simulink library "F_Line_block"  (R2018a)
settings: Solver=VariableStepAuto  StartTime=0.0  StopTime=10.0  RelTol=1e-3  EnableMultiTasking=on
settings Model: Creator=altari  LastModifiedBy=DW
settings DataIOCC: LimitDataPoints=on
settings OptimizationCC: LifeSpan=inf
settings DebuggingCC: AllowSymbolicDim=off  SFUnexpectedBacktrackingDiag=warning  SFNoUnconditionalDefaultTransitionDiag=warning  SFExecutionAtInitializationDiag=none
settings ModelReferenceCC: PropagateSignalLabelsOutOfModel=off
settings CodeAppCC: StateflowObjectComments=on
settings GRTTargetCC: TargetLangStandard=C89/C90 (ANSI)
settings ConfigComp: CovMetricSettings=dw  CovHtmlReporting=on  CovSaveCumulativeToWorkspaceVar=on  CovSaveSingleToWorkspaceVar=on  CovExternalEMLEnable=off

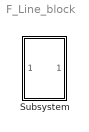
== system F_Line_block ==
  Subsystem : Subsystem

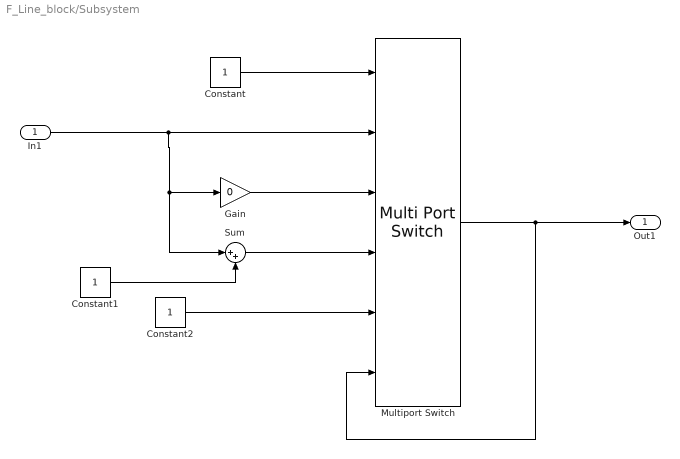
== system F_Line_block/Subsystem ==
  In1 : Inport
  Constant : Constant
  Constant1 : Constant
  Constant2 : Constant
  Gain : Gain  Gain=0
  Multiport Switch : MultiPortSwitch  Inputs=5
  Sum : Sum  Inputs=|++
  Out1 : Outport
  wires:
  Gain/1 -> Multiport Switch/3
  Constant/1 -> Multiport Switch/1
  Constant1/1 -> Sum/2
  Sum/1 -> Multiport Switch/4
  In1/1 -> Sum/1, Gain/1, Multiport Switch/2
  Multiport Switch/1 -> Out1/1, Multiport Switch/6
  Constant2/1 -> Multiport Switch/5
